simulink model "Drosselventil"  (R2021a)
settings: Solver=VariableStepAuto  StartTime=0.0  StopTime=10.0  RelTol=1e-3
settings Model: Creator=kbhan  LastModifiedBy=kbhan

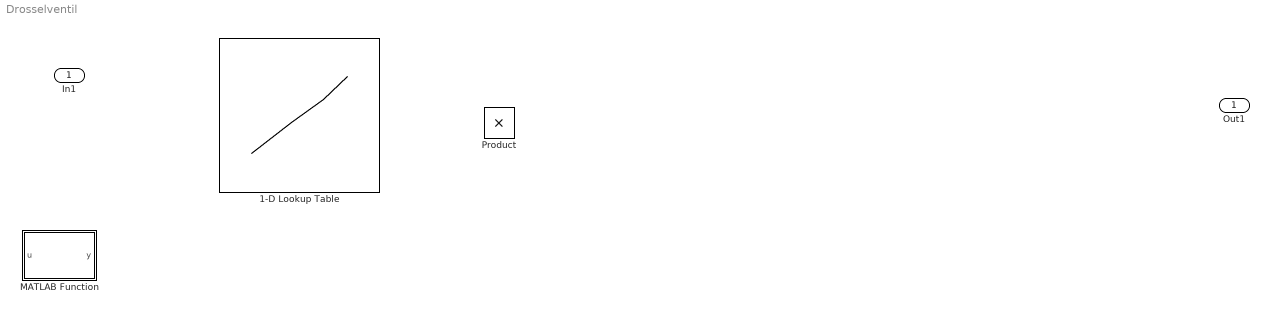
== system Drosselventil ==
  In1 : Inport
  1-D Lookup Table : Lookup_n-D  NumberOfTableDimensions=1  BreakpointsForDimension1=[0 0.05 0.1 0.15 0.2 0.25 0.3 0.35 0.4 0.45 0.5]  Table=[0 0.001 0.003 0.005 0.008 0.012 0.017 0.022 0.03 0.039 0.05]  InternalRulePriority=Speed  RndMeth=Simplest  InputSameDT=on
  MATLAB Function : MATLAB Function  TreatAsAtomicUnit=on
  Product : Product
  Out1 : Outport

== matlab function Drosselventil/MATLAB Function ==
  data: u input; y output
function y = fcn(u)
y = 10*u*(u<0.3)*(u>=0)+(10*u^1.8+1.85)*(u>=0.3);
